simulink model "Falownik_polmosek_polokresowa"  (R2022a)
settings: Solver=VariableStepAuto  StartTime=0.0  StopTime=300e-6  FixedStep=1e-9  RelTol=1e-3
libraries: spsSeriesRLCBranchLib x5, spsMosfetLib x2, spsOnDelayLib x2, spsVoltageMeasurementLib x2, spsCurrentMeasurementLib x1, spsDCVoltageSourceLib x1, spspowerguiLib x1
settings Model: Creator=szymo  LastModifiedBy=szymo

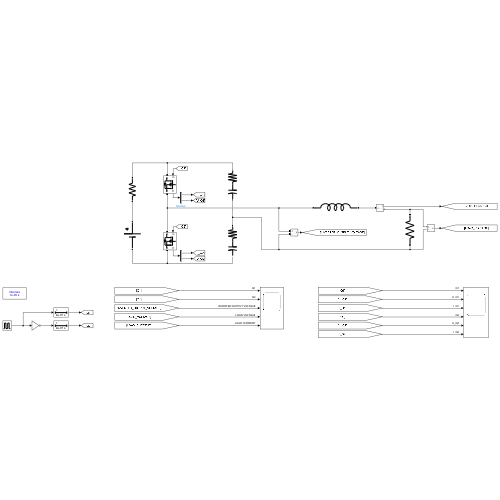
[thumbnail: Simulink's stored preview of the top-level diagram]
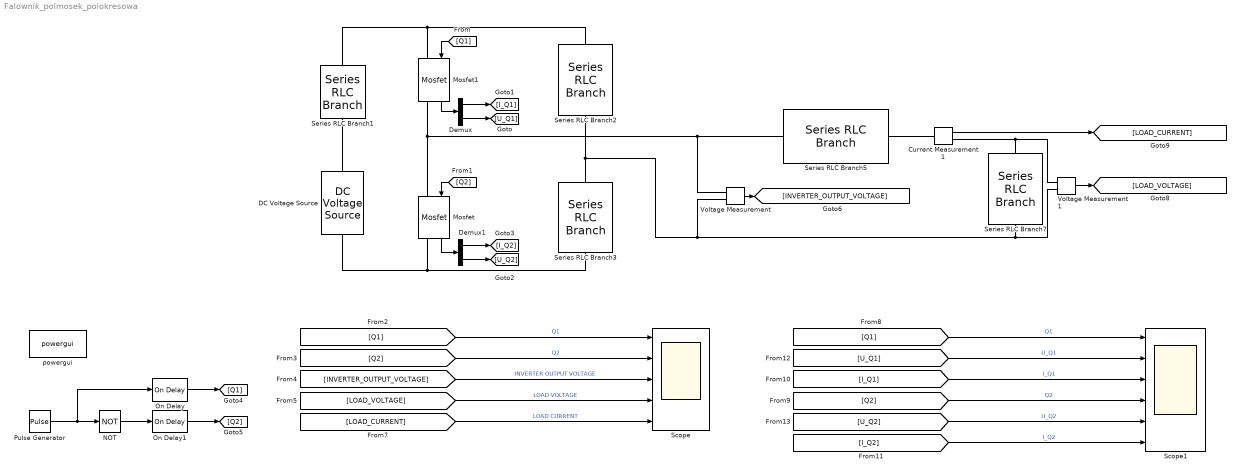
== system Falownik_polmosek_polokresowa ==
  Current Measurement1 : spsCurrentMeasurementLib/Current Measurement  PhasorSimulation=off  OutputType=Complex  PSBequivalent=0
  DC Voltage Source : spsDCVoltageSourceLib/DC Voltage Source  Amplitude=15  Measurements=None
  Demux : Demux  Outputs=2
  Demux1 : Demux  Outputs=2
  Mosfet : spsMosfetLib/Mosfet  Ron=20e-3  Lon=0  Rd=40e-3  Vfd=1  IC=0  Rs=1e5  Cs=inf  Measurements=on
  Mosfet1 : spsMosfetLib/Mosfet  Ron=20e-3  Lon=0  Rd=40e-3  Vfd=1  IC=0  Rs=1e5  Cs=inf  Measurements=on
  NOT : Logic  Operator=NOT  IconShape=distinctive  AllPortsSameDT=off  OutDataTypeStr=boolean
  On Delay : spsOnDelayLib/On Delay  DelayType=On delay  delay=200e-9  ic=0  Ts=0
      settings: SourceProductBaseCode=PS
  On Delay1 : spsOnDelayLib/On Delay  DelayType=On delay  delay=200e-9  ic=0  Ts=0
      settings: SourceProductBaseCode=PS
  Pulse Generator : DiscretePulseGenerator  PulseType=Time based  Period=1/10e3  PulseWidth=50
  Scope : Scope  NumInputPorts=5
  Scope1 : Scope  NumInputPorts=6
  Series RLC Branch1 : spsSeriesRLCBranchLib/Series RLC Branch  LConnTagsString=__new0  RConnTagsString=__new0  BranchType=R  Resistance=100e-3  Inductance=1e-3  SetiL0=off  InitialCurrent=0  Capacitance=1e-3  Setx0=on  InitialVoltage=400  Measurements=None
  Series RLC Branch2 : spsSeriesRLCBranchLib/Series RLC Branch  LConnTagsString=__new0  RConnTagsString=__new0  BranchType=RC  Resistance=10e-3  Inductance=1e-3  SetiL0=off  InitialCurrent=0  Capacitance=47e-6  Setx0=on  InitialVoltage=7.5  Measurements=None
  Series RLC Branch3 : spsSeriesRLCBranchLib/Series RLC Branch  LConnTagsString=__new0  RConnTagsString=__new0  BranchType=RC  Resistance=10e-3  Inductance=1e-3  SetiL0=off  InitialCurrent=0  Capacitance=47e-6  Setx0=on  InitialVoltage=7.5  Measurements=None
  Series RLC Branch5 : spsSeriesRLCBranchLib/Series RLC Branch  LConnTagsString=__new0  RConnTagsString=__new0  BranchType=L  Resistance=35e-3  Inductance=4e-6  SetiL0=off  InitialCurrent=0  Capacitance=470e-6  Setx0=on  InitialVoltage=200  Measurements=None
  Series RLC Branch7 : spsSeriesRLCBranchLib/Series RLC Branch  LConnTagsString=__new0  RConnTagsString=__new0  BranchType=R  Resistance=200  Inductance=1e-3  SetiL0=off  InitialCurrent=0  Capacitance=470e-6  Setx0=on  InitialVoltage=200  Measurements=None
  Voltage Measurement : spsVoltageMeasurementLib/Voltage Measurement  PhasorSimulation=off  OutputType=Complex  PSBequivalent=0
  Voltage Measurement1 : spsVoltageMeasurementLib/Voltage Measurement  PhasorSimulation=off  OutputType=Complex  PSBequivalent=0
  powergui : spspowerguiLib/powergui  Priority=1  SimulationMode=Discrete  SampleTime=1e-9  frequency=60  Iterations=50  frequencyindice=0  Pbase=100e6  ErrMax=1e-4  UnitsV=kV  UnitsW=MW  buscounter=0  FunctionMessages=off  echomessages=off  EnableUseOfTLC=off  CurrentSourceSwitches=off  DisableSnubberDevices=off  DisableRonSwitches=off  DisableVfSwitches=off  DisplayEquations=off  AutomaticDiscreteSolvers=off  SolverType=Tustin/Backward Euler (TBE)  Interpol=off  ExternalGateDelay=off  methode=off  Ts=100  x0status=blocks  SPID=on  SwTol=0  HookPort=off  NonlinearTolerance=1e-4  nMaxIteration=100  ContinueOnMaxIteration=off  RestoreLinks=warning  ResistiveCurrentMeasurement=off  Frange=[0:2:500]  Ylog=off  Xlog=on  ShowGrid=off  save=off  variable=ZData  structure=0  ZoomFFT=off  StartTime=0.0  cycles=1  DisplayStyle=1  fundamental=60  FreqAxis=off  MaxFrequency=1000  frequencyindicesteady=1  RmsSteady=1  display=off
  wires:
  [Q1] -> Mosfet1/1
  [Q2] -> Mosfet/1
  Mosfet1/1 -> Demux/1
  Mosfet/1 -> Demux1/1
  Pulse Generator/1 -> On Delay/1, NOT/1
  NOT/1 -> On Delay1/1
  On Delay/1 -> [Q1]
  On Delay1/1 -> [Q2]
  [Q1] -> Scope/1  "Q1"
  [Q2] -> Scope/2  "Q2"
  [INVERTER_OUTPUT_VOLTAGE] -> Scope/3  "INVERTER OUTPUT VOLTAGE"
  [LOAD_VOLTAGE] -> Scope/4  "LOAD VOLTAGE"
  [LOAD_CURRENT] -> Scope/5  "LOAD CURRENT"
  [Q2] -> Scope1/4  "Q2"
  [U_Q1] -> Scope1/2  "U_Q1"
  [I_Q1] -> Scope1/3  "I_Q1"
  [U_Q2] -> Scope1/5  "U_Q2"
  [I_Q2] -> Scope1/6  "I_Q2"
  [Q1] -> Scope1/1  "Q1"
  Voltage Measurement/1 -> [INVERTER_OUTPUT_VOLTAGE]
  Voltage Measurement1/1 -> [LOAD_VOLTAGE]
  Current Measurement1/1 -> [LOAD_CURRENT]
  Demux1/1 -> [I_Q2]
  Demux1/2 -> [U_Q2]
  Demux/2 -> [U_Q1]
  Demux/1 -> [I_Q1]
  connections:
  Mosfet1/RConn1 -- Voltage Measurement/LConn1 -- Series RLC Branch5/LConn1 -- Mosfet/LConn1
  DC Voltage Source/RConn1 -- Series RLC Branch1/RConn1
  DC Voltage Source/LConn1 -- Mosfet/RConn1 -- Series RLC Branch3/RConn1
  Series RLC Branch2/RConn1 -- Series RLC Branch3/LConn1 -- Voltage Measurement1/LConn2 -- Series RLC Branch7/RConn1 -- Voltage Measurement/LConn2
  Current Measurement1/LConn1 -- Series RLC Branch5/RConn1
  Current Measurement1/RConn1 -- Series RLC Branch7/LConn1 -- Voltage Measurement1/LConn1
  Series RLC Branch1/LConn1 -- Series RLC Branch2/LConn1 -- Mosfet1/LConn1
